simulink model "sim_generateur_gaz"  (Simulink 7.9)
settings: Solver=ode45  StartTime=0.0  StopTime=10.0  RelTol=1e-3
values from neighbouring files (symbols this model uses):
  ig = 0.086    [donnees_et_modeles_lineaires.mat]    (also in donnees_turbine_v2007a.mat)
  isong = [20000 21000 22000 23000 24000 25000 26000 27000 28000 29000 30000 31000 ... (16 elements, 16x1)]    [donnees_et_modeles_lineaires.mat]    (also in donnees_turbine_v2007a.mat)
  isowf = [40 80 120 160 200 240 280 320 360 400 440 480 ... (15 elements, 15x1)]    [donnees_et_modeles_lineaires.mat]    (also in donnees_turbine_v2007a.mat)
  itot = 0.250471468144    [donnees_et_modeles_lineaires.mat]    (also in donnees_turbine_v2007a.mat)
  ntlnom = 22800    [donnees_et_modeles_lineaires.mat]    (also in donnees_turbine_v2007a.mat)
  tcg = [-4.72566699982 -2.1958899498 0.325212001801 2.65510463715 5.70554542542 9.11180782318 12.5180749893 15.9243402481 19.3306007385 22.7368736267 26.1431350708 29.5494003296 ... (240 elements, 15x16)]    [donnees_et_modeles_lineaires.mat]    (also in donnees_turbine_v2007a.mat)
  tctl100 = [-0.0806421041489 -0.00261628627777 0.383603572845 0.214125156403 0.554617404938 0.27828836441 0.00195932388306 -0.274368286133 -0.55069732666 -0.827028751373 -1.10335540771 -1.37968444824 ... (240 elements, 15x16)]    [donnees_et_modeles_lineaires.mat]    (also in donnees_turbine_v2007a.mat)
  tdctldntl = [-0.000853070175439 -0.000853070175439 -0.000853070175439 -0.000853070175439 -0.00046798245614 -0.00101842105263 -0.0012701754386 -0.00134210526316 -0.00138728070175 -0.00140219298246 -0.00144561403509 -0.00155526315789 ... (16 elements, 16x1)]    [donnees_et_modeles_lineaires.mat]    (also in donnees_turbine_v2007a.mat)
  tdos = 0.054    [donnees_et_modeles_lineaires.mat]    (also in donnees_turbine_v2007a.mat)
  tp3 = [1.74359560013 1.83476543427 1.89652109146 1.97084283829 2.02915382385 2.07755017281 2.12594628334 2.17434239388 2.22273850441 2.27113461494 2.31953167915 2.36792778969 ... (240 elements, 15x16)]    [donnees_et_modeles_lineaires.mat]    (also in donnees_turbine_v2007a.mat)
  tt4 = [158.323181152 257.927246094 378.081359863 509.409484863 632.046447754 753.55480957 875.063598633 996.572021484 1118.07995605 1239.58874512 1361.09716797 1482.60595703 ... (240 elements, 15x16)]    [donnees_et_modeles_lineaires.mat]    (also in donnees_turbine_v2007a.mat)
  tth = 0.8    [donnees_et_modeles_lineaires.mat]    (also in donnees_turbine_v2007a.mat)
settings Model: Creator=maffre  LastModifiedBy=maffre

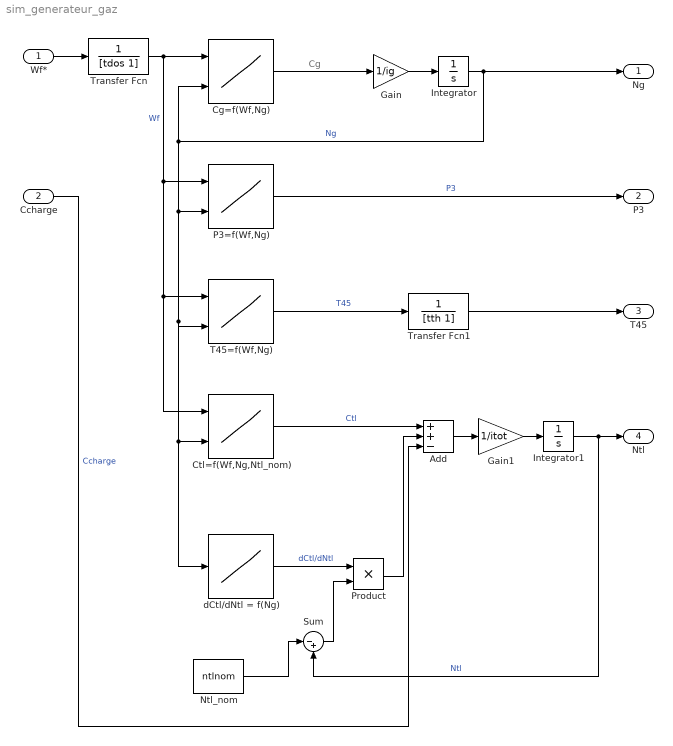
== system sim_generateur_gaz ==
  note: Cg
  Wf* : Inport
  Ccharge : Inport  Port=2
  Add : Sum  Inputs=++-
  Cg=f(Wf,Ng) : Lookup_n-D  BreakpointsForDimension1=isowf  BreakpointsForDimension2=isong  Table=tcg  RndMeth=Simplest  InputSameDT=on
  Ctl=f(Wf,Ng,Ntl_nom) : Lookup_n-D  BreakpointsForDimension1=isowf  BreakpointsForDimension2=isong  Table=tctl100  RndMeth=Simplest  InputSameDT=on
  Gain : Gain  Gain=1/ig
  Gain1 : Gain  Gain=1/itot
  Integrator : Integrator
  Integrator1 : Integrator
  Ntl_nom : Constant  Value=ntlnom
  P3=f(Wf,Ng) : Lookup_n-D  BreakpointsForDimension1=isowf  BreakpointsForDimension2=isong  Table=tp3  RndMeth=Simplest  InputSameDT=on
  Product : Product  RndMeth=Zero
  Sum : Sum  Inputs=|-+
  T45=f(Wf,Ng) : Lookup_n-D  BreakpointsForDimension1=isowf  BreakpointsForDimension2=isong  Table=tt4  RndMeth=Simplest  InputSameDT=on
  Transfer Fcn : TransferFcn  Denominator=[tdos 1]
  Transfer Fcn1 : TransferFcn  Denominator=[tth 1]
  dCtl/dNtl = f(Ng) : Lookup_n-D  NumberOfTableDimensions=1  BreakpointsForDimension1=isong  Table=tdctldntl  RndMeth=Simplest  InputSameDT=on
  Ng : Outport
  P3 : Outport  Port=2
  T45 : Outport  Port=3
  Ntl : Outport  Port=4
  wires:
  Transfer Fcn1/1 -> T45/1
  Integrator/1 -> Ng/1, Cg=f(Wf,Ng)/2, P3=f(Wf,Ng)/2, T45=f(Wf,Ng)/2, Ctl=f(Wf,Ng,Ntl_nom)/2, dCtl/dNtl = f(Ng)/1  "Ng"
  Gain/1 -> Integrator/1
  Cg=f(Wf,Ng)/1 -> Gain/1
  Wf*/1 -> Transfer Fcn/1
  Transfer Fcn/1 -> Cg=f(Wf,Ng)/1, P3=f(Wf,Ng)/1, T45=f(Wf,Ng)/1, Ctl=f(Wf,Ng,Ntl_nom)/1  "Wf"
  P3=f(Wf,Ng)/1 -> P3/1  "P3"
  T45=f(Wf,Ng)/1 -> Transfer Fcn1/1  "T45"
  dCtl/dNtl = f(Ng)/1 -> Product/1  "dCtl/dNtl"
  Sum/1 -> Product/2
  Ctl=f(Wf,Ng,Ntl_nom)/1 -> Add/1  "Ctl"
  Product/1 -> Add/2
  Gain1/1 -> Integrator1/1
  Integrator1/1 -> Ntl/1, Sum/2  "Ntl"
  Add/1 -> Gain1/1
  Ntl_nom/1 -> Sum/1
  Ccharge/1 -> Add/3  "Ccharge"
